simulink model "L02_TrafficLightController"  (R2021a)
settings: Solver=FixedStepDiscrete  StartTime=0.0  StopTime=120.0  FixedStep=0.1  RelTol=1e-3
settings Model: EnablePacing=on  PacingRate=6  Creator=ncleju  LastModifiedBy=Nic

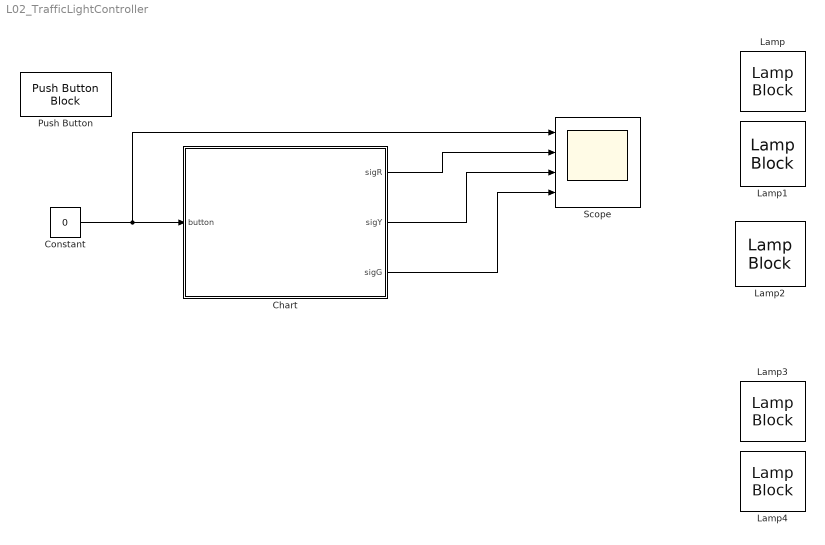
== system L02_TrafficLightController ==
  Chart : Stateflow chart  TreatAsAtomicUnit=on
  Constant : Constant  Value=0
  Lamp{,1..4} (5 alike) : LampBlock
  Push Button : PushButtonBlock
  Scope : Scope  NumInputPorts=4
  wires:
  Constant/1 -> Scope/1, Chart/1(button)
  Chart/1(sigR) -> Scope/2
  Chart/2(sigY) -> Scope/3
  Chart/3(sigG) -> Scope/4

== stateflow chart L02_TrafficLightController/Chart ==
  state YELLOW
    entry:
    sigR=false;
    sigY=true;
    sigG=false;
  state RED
    entry:
    sigR=true;
    sigY=false;
    sigG=false;
  state GREEN
    entry:
    sigR=false;
    sigY=false;
    sigG=true;
  (default) -> RED
  YELLOW -> RED : [after(50, tick)]
  RED -> GREEN : [after(30, sec)]
      | {count = 0;
      | pressed = false;}
  GREEN -> YELLOW [order 1] : [(pressed== true) && (count >= 600)]
  GREEN -> GREEN [order 2] : [button == true]
      | {pressed = true;
      | count = count+1;}
  GREEN -> GREEN [order 3] : {count = count+1;}
  data: button input; sigR output; sigY output; count local; sigG output; pressed local
